simulink model "Preview_stanley"  (R2021a)
settings: configuration reference "AION_IDS_Speedgoat" (kept outside this file)
libraries: simulink_extras x2, simulink x1
settings Model: DataDictionary=Preview_Stanley.sldd  Creator=xinrui  LastModifiedBy=Administrator
settings ConfigSetRef: SourceName=AION_IDS_Speedgoat

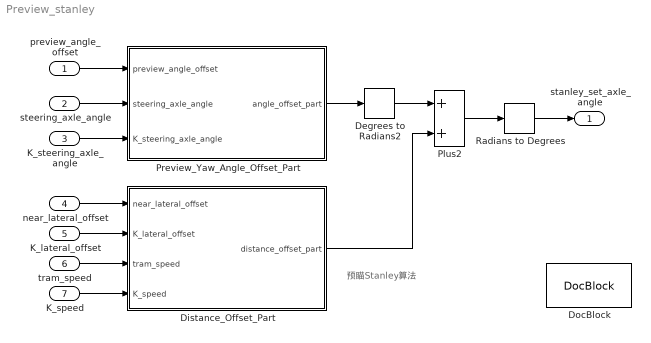
== system Preview_stanley ==
  note: 预瞄Stanley算法
  preview_angle_offset : Inport  OutDataTypeStr=double  PortDimensions=1
  steering_axle_angle : Inport  Port=2  OutDataTypeStr=double  PortDimensions=1
  K_steering_axle_angle : Inport  Port=3  OutDataTypeStr=double  PortDimensions=1
  near_lateral_offset : Inport  Port=4  OutDataTypeStr=double  PortDimensions=1
  K_lateral_offset : Inport  Port=5  OutDataTypeStr=double  PortDimensions=1
  tram_speed : Inport  Port=6  OutDataTypeStr=double  PortDimensions=1
  K_speed : Inport  Port=7  OutDataTypeStr=double  PortDimensions=1
  Degrees to Radians2 : simulink_extras/Transformations/Degrees to Radians
  Distance_Offset_Part : Subsystem
  DocBlock : simulink/Model-Wide Utilities/DocBlock  DocumentType=HTML  mask(DocBlock){}
      mask Display:
      | plot([.8 0 0 1 1 .8 .8 1],[1 1 0 0 .8 1 .8 .8]);
      | text(.5,.6,'CHANGELOG','horizontalalignment','center');
      | text(.95,.05,get_param(gcb,'DocumentType'),'verticalalignment','bottom','horizontalalignment','right');
  Plus2 : Sum  OutDataTypeStr=double
  Preview_Yaw_Angle_Offset_Part : Subsystem
  Radians to Degrees : simulink_extras/Transformations/Radians to Degrees
  stanley_set_axle_angle : Outport  OutDataTypeStr=double  PortDimensions=1
  wires:
  near_lateral_offset/1 -> Distance_Offset_Part/1(near_lateral_offset)
  Plus2/1 -> Radians to Degrees/1
  preview_angle_offset/1 -> Preview_Yaw_Angle_Offset_Part/1(preview_angle_offset)
  Distance_Offset_Part/1(distance_offset_part) -> Plus2/2
  K_speed/1 -> Distance_Offset_Part/4(K_speed)
  K_lateral_offset/1 -> Distance_Offset_Part/2(K_lateral_offset)
  Preview_Yaw_Angle_Offset_Part/1(angle_offset_part) -> Degrees to Radians2/1
  tram_speed/1 -> Distance_Offset_Part/3(tram_speed)
  steering_axle_angle/1 -> Preview_Yaw_Angle_Offset_Part/2(steering_axle_angle)
  Radians to Degrees/1 -> stanley_set_axle_angle/1
  K_steering_axle_angle/1 -> Preview_Yaw_Angle_Offset_Part/3(K_steering_axle_angle)
  Degrees to Radians2/1 -> Plus2/1

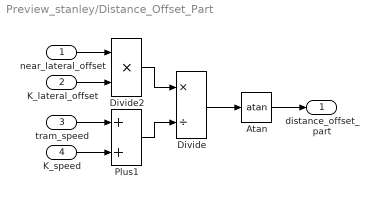
== system Preview_stanley/Distance_Offset_Part ==
  near_lateral_offset : Inport  OutDataTypeStr=double  PortDimensions=1
  K_lateral_offset : Inport  Port=2  OutDataTypeStr=double  PortDimensions=1
  tram_speed : Inport  Port=3  OutDataTypeStr=double  PortDimensions=1
  K_speed : Inport  Port=4  OutDataTypeStr=double  PortDimensions=1
  Atan : Trigonometry  Operator=atan  OutputSignalType=real
  Divide : Product  Inputs=*/  OutDataTypeStr=double
  Divide2 : Product  Inputs=**  OutDataTypeStr=double
  Plus1 : Sum  OutDataTypeStr=double
  distance_offset_part : Outport  OutDataTypeStr=double  PortDimensions=1
  wires:
  near_lateral_offset/1 -> Divide2/1
  K_lateral_offset/1 -> Divide2/2
  Atan/1 -> distance_offset_part/1
  Plus1/1 -> Divide/2
  tram_speed/1 -> Plus1/1
  K_speed/1 -> Plus1/2
  Divide/1 -> Atan/1
  Divide2/1 -> Divide/1

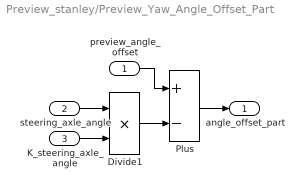
== system Preview_stanley/Preview_Yaw_Angle_Offset_Part ==
  preview_angle_offset : Inport  OutDataTypeStr=double  PortDimensions=1
  steering_axle_angle : Inport  Port=2  OutDataTypeStr=double  PortDimensions=1
  K_steering_axle_angle : Inport  Port=3  OutDataTypeStr=double  PortDimensions=1
  Divide1 : Product  Inputs=**  OutDataTypeStr=double
  Plus : Sum  Inputs=+-  OutDataTypeStr=double
  angle_offset_part : Outport  OutDataTypeStr=double  PortDimensions=1
  wires:
  steering_axle_angle/1 -> Divide1/1
  Plus/1 -> angle_offset_part/1
  preview_angle_offset/1 -> Plus/1
  K_steering_axle_angle/1 -> Divide1/2
  Divide1/1 -> Plus/2
